simulink model "Quadrotor_two_blocks"  (R2020a)
settings: Solver=FixedStepAuto  StartTime=0.0  StopTime=options.T_train  FixedStep=options.dt  RelTol=1e-6
undefined symbols (not defined in the file or in its folder): options, Quad
libraries: neural x205, simulink x3
(part 11 of 14)

== system Quadrotor_two_blocks/NN_cex_1/Layer 3/Delays 1 ==
  "p{3}" : Inport  PortDimensions=30
      mask Display: e = 0.06;c1 = [120 230 180]/255;c2 = ([120 230 180]+0)/(256+128);c3 = ([120 230 180]+128)/(256+128);patch([0 1 1 0],[0 0 1 1],c1);patch([0 1 1 1-e 1-e 0+e],[0 0 1 1-e 0+e 0+e],c2);patch([0 0 1 1-e 0+e 0+e],[0 1 1 1-e 1-e 0+e],c3);plot([0 1 1 0 0],[0 0 1 1 0]);
  mux : Mux  Inputs=1
      mask Display: e = 0.06;c1 = [120 150 230]/255;c2 = ([120 150 230]+0)/383;c3 = ([120 150 230]+128)/383;patch([0 1 1 0],[0 0 1 1],c1);patch([0 1 1 1-e 1-e 0+e],[0 0 1 1-e 0+e 0+e],c2);patch([0 0 1 1-e 0+e 0+e],[0 1 1 1-e 1-e 0+e],c3);plot([0 1 1 0 0],[0 0 1 1 0]);disp('Mux')
  "pd{3,2}" : Outport
      mask Display: e = 0.06;c1 = [120 230 180]/255;c2 = ([120 230 180]+0)/(256+128);c3 = ([120 230 180]+128)/(256+128);patch([0 1 1 0],[0 0 1 1],c1);patch([0 1 1 1-e 1-e 0+e],[0 0 1 1-e 0+e 0+e],c2);patch([0 0 1 1-e 0+e 0+e],[0 1 1 1-e 1-e 0+e],c3);plot([0 1 1 0 0],[0 0 1 1 0]);
  wires:
  "p{3}"/1 -> mux/1
  mux/1 -> "pd{3,2}"/1

== system Quadrotor_two_blocks/NN_cex_1/Layer 3/LW{3,2} ==
  "ad{3,2}" : Inport  PortDimensions=30
      mask Display: e = 0.06;c1 = [120 230 180]/255;c2 = ([120 230 180]+0)/(256+128);c3 = ([120 230 180]+128)/(256+128);patch([0 1 1 0],[0 0 1 1],c1);patch([0 1 1 1-e 1-e 0+e],[0 0 1 1-e 0+e 0+e],c2);patch([0 0 1 1-e 0+e 0+e],[0 1 1 1-e 1-e 0+e],c3);plot([0 1 1 0 0],[0 0 1 1 0]);
  "IW{3,2}(1,:)'" : Constant  Value=[-0.58128505172544198131845405441708862781524658203125;-0.2293273101975140948471931778840371407568454742431640625;0.21685369095220174973093207881902344524860382080078125;0.10477741850031456471992186152419890277087688446044921875;-0.2132629575955962142330690767266787588596343994140625;-0.32810670423877408286017498539877124130725860595703125;-0.79366274179956752821141208187327720224857330322265625;-0.8745625211368246443299767634016461670398712158203125;-0.170332859903608524465568052619346417486667633056640625;0.446676693703509375410476422985084354877471923828125;0.190618303720598569750421802382334135472774505615234375;0.3473696685972160747013504078495316207408905029296875;0.38339970252730370958715866436250507831573486328125;0.4623931517073451846755460792337544262409210205078125;-0.052959469136107474585006826828248449601233005523681640625;-0.68460079171598520186847736113122664391994476318359375;-0.570400321025498868721115286462008953094482421875;0.864929840758637435982336683082394301891326904296875;0.09021107685018119048958595840304042212665081024169921875;0.54343728966987081552275640206062234938144683837890625;0.50760133236115290156220680728438310325145721435546875;0.3434852528420180295398722591926343739032745361328125;0.061734581640343212660670957347974763251841068267822265625;-0.59774440960589025895188797221635468304157257080078125;0.52123091755720796225404001233982853591442108154296875;-0.52122498935737027192516279683331958949565887451171875;0.11177025658208324110365339265626971609890460968017578125;-0.517681742435928793355515153962187469005584716796875;0.03623388390739368247750462614931166172027587890625;0.09968869080000276883257726012743660248816013336181640625]
      mask Display: e = 0.06;c1 = [120 150 230]/255;c2 = ([120 150 230]+0)/383;c3 = ([120 150 230]+128)/383;patch([0 1 1 0],[0 0 1 1],c1);patch([0 1 1 1-e 1-e 0+e],[0 0 1 1-e 0+e 0+e],c2);patch([0 0 1 1-e 0+e 0+e],[0 1 1 1-e 1-e 0+e],c3);plot([0 1 1 0 0],[0 0 1 1 0]);disp('weights');
  "IW{3,2}(2,:)'" : Constant  Value=[0.6300025847661816502665033112862147390842437744140625;0.24662395119319946434899293308262713253498077392578125;0.35122330596911333078224970449809916317462921142578125;-0.224613954967990803179844760961714200675487518310546875;0.5453869849357284582680449602776207029819488525390625;0.7279480611954858293444203809485770761966705322265625;-0.266598090960109390668009154978790320456027984619140625;0.01194367017760886683086507531470488174818456172943115234375;-0.31999494149323137737184197249007411301136016845703125;-0.42856324948409107999935940824798308312892913818359375;-0.231652605048332571602287544010323472321033477783203125;-0.289561248087723821509342769786599092185497283935546875;0.60662774498312865834037665990763343870639801025390625;0.48860144164990126913750145831727422773838043212890625;-0.79637255744750723440716910772607661783695220947265625;0.675314808226324725382028191233985126018524169921875;-0.386247503858614338323462789048790000379085540771484375;0.040632618405469000943952551097027026116847991943359375;0.32523619769138278901010608024080283939838409423828125;0.70784847926255956007679515096242539584636688232421875;-0.76955599959751108674055330993724055588245391845703125;-0.68896605044519410032677342314855195581912994384765625;-0.499800292110237076581569226618739776313304901123046875;-0.85350006671610489927815024202573113143444061279296875;0.7096144101352142019578650433686561882495880126953125;0.387011282028088710038815634106867946684360504150390625;0.6415290925225638485329682225710712373256683349609375;-0.2058035886973335892857761564300744794309139251708984375;-0.2598073416204658148132011774578131735324859619140625;0.09915147768814502882150918594561517238616943359375]
      mask Display: e = 0.06;c1 = [120 150 230]/255;c2 = ([120 150 230]+0)/383;c3 = ([120 150 230]+128)/383;patch([0 1 1 0],[0 0 1 1],c1);patch([0 1 1 1-e 1-e 0+e],[0 0 1 1-e 0+e 0+e],c2);patch([0 0 1 1-e 0+e 0+e],[0 1 1 1-e 1-e 0+e],c3);plot([0 1 1 0 0],[0 0 1 1 0]);disp('weights');
  "IW{3,2}(3,:)'" : Constant  Value=[0.316944853432273132565200057797483168542385101318359375;0.8536006236562017068791874407907016575336456298828125;0.80176926909032764090312639382318593561649322509765625;0.3237126474993974323268730586278252303600311279296875;-0.32208997972446240520838500742684118449687957763671875;0.339696648877345352968148972649942152202129364013671875;0.43365464213477700194943054157192818820476531982421875;0.542662787313724859217245466425083577632904052734375;-0.859641875046941894566998598747886717319488525390625;-0.7896295765640000130503040054463781416416168212890625;0.1802415594194312353781839419752941466867923736572265625;-0.7122856402475452597400362719781696796417236328125;1.015639256722380423525464721024036407470703125;0.6565525957520852440296721397317014634609222412109375;0.23748238638691498980648475480847992002964019775390625;-0.7791592768606447894086386440903879702091217041015625;0.36785133107586276413059067635913379490375518798828125;0.349505691106954063940293053747154772281646728515625;0.6213517445924452431427198462188243865966796875;-0.69841255457959139363310896442271769046783447265625;-0.032322242612540109940599819537965231575071811676025390625;0.4408201050880522497976699014543555676937103271484375;-0.84263125440752972838964751645107753574848175048828125;-0.64619496494892547655553016738849692046642303466796875;-0.031594494162081161736654877358887461014091968536376953125;0.409865599114647427558821846105274744331836700439453125;0.2043849554957174741165459863623254932463169097900390625;0.60692013619355533737831365215242840349674224853515625;0.320703787806943474425480644640629179775714874267578125;-0.1841764905849182787367368518971488811075687408447265625]
      mask Display: e = 0.06;c1 = [120 150 230]/255;c2 = ([120 150 230]+0)/383;c3 = ([120 150 230]+128)/383;patch([0 1 1 0],[0 0 1 1],c1);patch([0 1 1 1-e 1-e 0+e],[0 0 1 1-e 0+e 0+e],c2);patch([0 0 1 1-e 0+e 0+e],[0 1 1 1-e 1-e 0+e],c3);plot([0 1 1 0 0],[0 0 1 1 0]);disp('weights');
  "IW{3,2}(4,:)'" : Constant  Value=[-0.73899685454495533942775864488794468343257904052734375;0.1329015978629735084126650690450333058834075927734375;-0.71245043248978967564966069403453730046749114990234375;0.78013232508547314392188809506478719413280487060546875;0.1637189859343445574868525227429927326738834381103515625;0.62178818385121470413423594436608254909515380859375;-0.52252035416292141878358279427629895508289337158203125;-0.342898521357951346910653001032187603414058685302734375;0.03126596413692618592339300676030688919126987457275390625;-0.52450888410719809229476595646701753139495849609375;-0.8761196704679379276825557099073193967342376708984375;-0.13585063293048793564565812630462460219860076904296875;0.995897036543297975441646485705859959125518798828125;0.162110102883930962125447194921434856951236724853515625;0.64305996304890544745802571924286894500255584716796875;-0.235993414328976081062450020908727310597896575927734375;-0.348571423291109627751183097643661312758922576904296875;-0.8971978321175431148049028706736862659454345703125;0.322772727228386069331378394053899683058261871337890625;-0.50343883079882412179273387664579786360263824462890625;-0.45078677028053848463429176263161934912204742431640625;0.55902820248842355344010002227150835096836090087890625;0.1996427857195924027156053170983796007931232452392578125;-0.01625974335785830560130449384814710356295108795166015625;-0.95004935805964141337653927621431648731231689453125;-0.482551033452830291370361237568431533873081207275390625;0.01394217697500968293489176375032911892049014568328857421875;-0.235723023430602862671179309472790919244289398193359375;0.08184667106743226394627299669082276523113250732421875;0.0190188442369213540905636961042546317912638187408447265625]
      mask Display: e = 0.06;c1 = [120 150 230]/255;c2 = ([120 150 230]+0)/383;c3 = ([120 150 230]+128)/383;patch([0 1 1 0],[0 0 1 1],c1);patch([0 1 1 1-e 1-e 0+e],[0 0 1 1-e 0+e 0+e],c2);patch([0 0 1 1-e 0+e 0+e],[0 1 1 1-e 1-e 0+e],c3);plot([0 1 1 0 0],[0 0 1 1 0]);disp('weights');
  Mux : Mux
      mask Display: e = 0.06;c1 = [120 150 230]/255;c2 = ([120 150 230]+0)/383;c3 = ([120 150 230]+128)/383;patch([0 1 1 0],[0 0 1 1],c1);patch([0 1 1 1-e 1-e 0+e],[0 0 1 1-e 0+e 0+e],c2);patch([0 0 1 1-e 0+e 0+e],[0 1 1 1-e 1-e 0+e],c3);plot([0 1 1 0 0],[0 0 1 1 0]);disp('Mux');
  dotprod{1..4} (4 alike) : neural/Weight Functions/dotprod
  "lz{3,2}" : Outport
      mask Display: e = 0.06;c1 = [120 230 180]/255;c2 = ([120 230 180]+0)/(256+128);c3 = ([120 230 180]+128)/(256+128);patch([0 1 1 0],[0 0 1 1],c1);patch([0 1 1 1-e 1-e 0+e],[0 0 1 1-e 0+e 0+e],c2);patch([0 0 1 1-e 0+e 0+e],[0 1 1 1-e 1-e 0+e],c3);plot([0 1 1 0 0],[0 0 1 1 0]);
  wires:
  "IW{3,2}(1,:)'"/1 -> dotprod1/1
  "ad{3,2}"/1 -> dotprod1/2, dotprod2/2, dotprod3/2, dotprod4/2
  dotprod1/1 -> Mux/1
  "IW{3,2}(2,:)'"/1 -> dotprod2/1
  dotprod2/1 -> Mux/2
  "IW{3,2}(3,:)'"/1 -> dotprod3/1
  dotprod3/1 -> Mux/3
  "IW{3,2}(4,:)'"/1 -> dotprod4/1
  dotprod4/1 -> Mux/4
  Mux/1 -> "lz{3,2}"/1

== system Quadrotor_two_blocks/NN_online/Layer 1/Delays 1 ==
  "p{1}" : Inport  PortDimensions=20
      mask Display: e = 0.06;c1 = [120 230 180]/255;c2 = ([120 230 180]+0)/(256+128);c3 = ([120 230 180]+128)/(256+128);patch([0 1 1 0],[0 0 1 1],c1);patch([0 1 1 1-e 1-e 0+e],[0 0 1 1-e 0+e 0+e],c2);patch([0 0 1 1-e 0+e 0+e],[0 1 1 1-e 1-e 0+e],c3);plot([0 1 1 0 0],[0 0 1 1 0]);
  mux : Mux  Inputs=1
      mask Display: e = 0.06;c1 = [120 150 230]/255;c2 = ([120 150 230]+0)/383;c3 = ([120 150 230]+128)/383;patch([0 1 1 0],[0 0 1 1],c1);patch([0 1 1 1-e 1-e 0+e],[0 0 1 1-e 0+e 0+e],c2);patch([0 0 1 1-e 0+e 0+e],[0 1 1 1-e 1-e 0+e],c3);plot([0 1 1 0 0],[0 0 1 1 0]);disp('Mux')
  "pd{1,1}" : Outport
      mask Display: e = 0.06;c1 = [120 230 180]/255;c2 = ([120 230 180]+0)/(256+128);c3 = ([120 230 180]+128)/(256+128);patch([0 1 1 0],[0 0 1 1],c1);patch([0 1 1 1-e 1-e 0+e],[0 0 1 1-e 0+e 0+e],c2);patch([0 0 1 1-e 0+e 0+e],[0 1 1 1-e 1-e 0+e],c3);plot([0 1 1 0 0],[0 0 1 1 0]);
  wires:
  "p{1}"/1 -> mux/1
  mux/1 -> "pd{1,1}"/1
